simulink model "constant_test"  (Simulink 8.4)
settings: Solver=ode45  StartTime=0.0  StopTime=10.0  RelTol=1e-3
settings Model: Creator=arnaud  LastModifiedBy=arnaud
settings DataIOCC: SaveFormat=Structure
settings DebuggingCC: StrictBusMsg=Warning

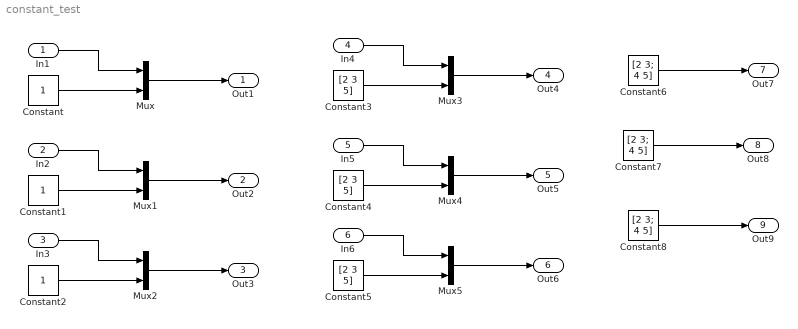
== system constant_test ==
  In1 : Inport  OutDataTypeStr=double
  In2 : Inport  Port=2  OutDataTypeStr=int8
  In3 : Inport  Port=3  OutDataTypeStr=boolean
  In4 : Inport  Port=4  OutDataTypeStr=double
  In5 : Inport  Port=5  OutDataTypeStr=int8
  In6 : Inport  Port=6  OutDataTypeStr=boolean
  Constant : Constant  OutDataTypeStr=double
  Constant1 : Constant  OutDataTypeStr=int8
  Constant2 : Constant  OutDataTypeStr=boolean
  Constant3 : Constant  Value=[2 3 5]  OutDataTypeStr=double
  Constant4 : Constant  Value=[2 3 5]  OutDataTypeStr=int8
  Constant5 : Constant  Value=[2 3 5]  OutDataTypeStr=boolean
  Constant6 : Constant  Value=[2 3; 4 5]  OutDataTypeStr=double
  Constant7 : Constant  Value=[2 3; 4 5]  OutDataTypeStr=int8
  Constant8 : Constant  Value=[2 3; 4 5]  OutDataTypeStr=boolean
  Mux{,1..5} (6 alike) : Mux  Inputs=2
  Out1 : Outport
  Out2 : Outport  Port=2
  Out3 : Outport  Port=3
  Out4 : Outport  Port=4
  Out5 : Outport  Port=5
  Out6 : Outport  Port=6
  Out7 : Outport  Port=7
  Out8 : Outport  Port=8
  Out9 : Outport  Port=9
  wires:
  In1/1 -> Mux/1
  Constant/1 -> Mux/2
  Mux/1 -> Out1/1
  In2/1 -> Mux1/1
  Constant1/1 -> Mux1/2
  Mux1/1 -> Out2/1
  In3/1 -> Mux2/1
  Constant2/1 -> Mux2/2
  Mux2/1 -> Out3/1
  In4/1 -> Mux3/1
  Constant3/1 -> Mux3/2
  Mux3/1 -> Out4/1
  In5/1 -> Mux4/1
  Constant4/1 -> Mux4/2
  Mux4/1 -> Out5/1
  In6/1 -> Mux5/1
  Constant5/1 -> Mux5/2
  Mux5/1 -> Out6/1
  Constant6/1 -> Out7/1
  Constant7/1 -> Out8/1
  Constant8/1 -> Out9/1
